simulink subsystem "s0330_swing_fast"  (R2019b)
settings: Solver=VariableStepAuto  StartTime=0.0  StopTime=10.0  RelTol=1e-3
settings Model: Creator=alessandro  LastModifiedBy=giaco

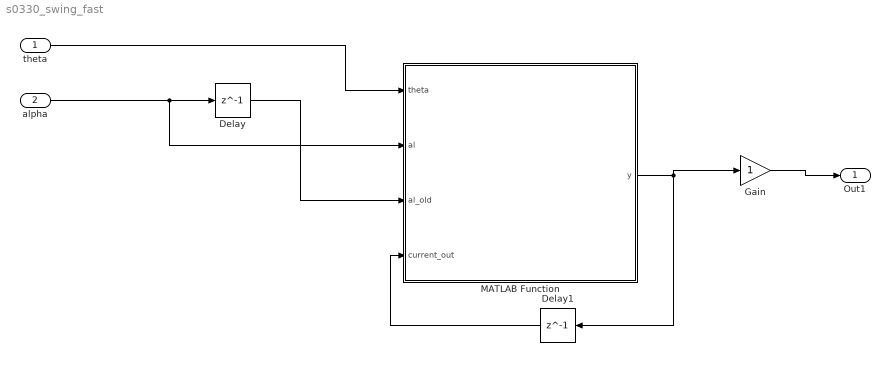
== system s0330_swing_fast ==
  theta : Inport
  alpha : Inport  Port=2
  Delay : Delay  DelayLength=1  InitialCondition=0
  Delay1 : Delay  DelayLength=1  InitialCondition=1
  Gain : Gain
  MATLAB Function : MATLAB Function  TreatAsAtomicUnit=on
  Out1 : Outport
  wires:
  theta/1 -> MATLAB Function/1(theta)
  alpha/1 -> MATLAB Function/2(al), Delay/1
  Gain/1 -> Out1/1
  Delay1/1 -> MATLAB Function/4(current_out)
  Delay/1 -> MATLAB Function/3(al_old)
  MATLAB Function/1(y) -> Gain/1, Delay1/1

== matlab function s0330_swing_fast/MATLAB Function ==
  data: theta input; y output; al input; al_old input; current_out input
function y = fcn(theta, al, al_old, current_out)
    if al < al_old && current_out == 1
        signum = -1;
    elseif al > al_old && current_out == -1
        signum = 1;
    else
        signum = sign(current_out);
    end
    
    mod = 5 - abs(theta)*(4/(pi/3));
    mod = max(mod, 1);  
y = signum*mod;
